simulink model "ex1"  (R2022a)
settings: Solver=VariableStepAuto  StartTime=0.0  StopTime=10.0  RelTol=1e-3
settings Model: Creator=loryb  LastModifiedBy=loryb

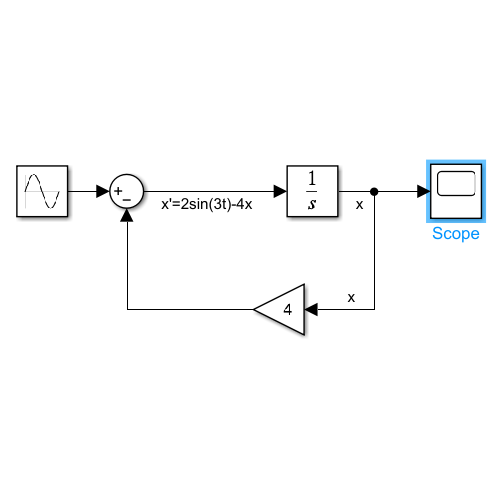
[thumbnail: Simulink's stored preview of the top-level diagram]
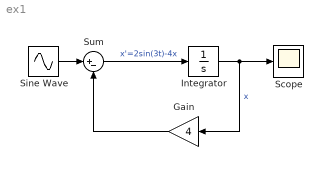
== system ex1 ==
  Gain : Gain  Gain=4
  Integrator : Integrator
  Scope : Scope
  Sine Wave : Sin  Amplitude=2  Frequency=3  SampleTime=0
  Sum : Sum  Inputs=|+-
  wires:
  Sine Wave/1 -> Sum/1
  Sum/1 -> Integrator/1  "x'=2sin(3t)-4x"
  Integrator/1 -> Gain/1, Scope/1  "x"
  Gain/1 -> Sum/2
